simulink model "MPC_variants"  (R2026a)
settings: Solver=FixedStepAuto
settings Model: Creator=rayyu  LastModifiedBy=rayyu
settings RTWCC: SystemTargetFile=ert.tlc  Description=Embedded Coder
settings ERTTargetCC: GenerateSampleERTMain=on

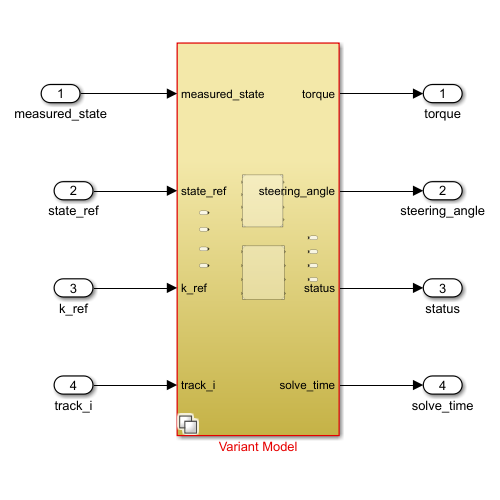
[thumbnail: Simulink's stored preview of the top-level diagram]
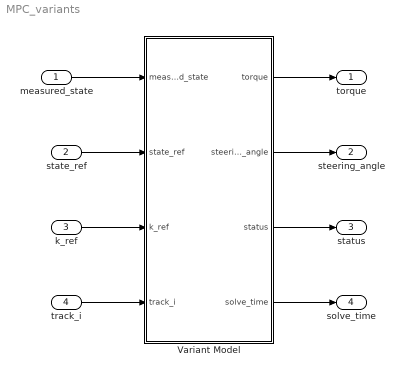
== system MPC_variants ==
  measured_state : Inport
  state_ref : Inport  Port=2
  k_ref : Inport  Port=3
  track_i : Inport  Port=4
  Variant Model : Subsystem  Variant=on
  torque : Outport
  steering_angle : Outport  Port=2
  status : Outport  Port=3
  solve_time : Outport  Port=4
  wires:
  measured_state/1 -> Variant Model/1(measured_state)
  state_ref/1 -> Variant Model/2(state_ref)
  k_ref/1 -> Variant Model/3(k_ref)
  track_i/1 -> Variant Model/4(track_i)
  Variant Model/1(torque) -> torque/1
  Variant Model/2(steering_angle) -> steering_angle/1
  Variant Model/3(status) -> status/1
  Variant Model/4(solve_time) -> solve_time/1

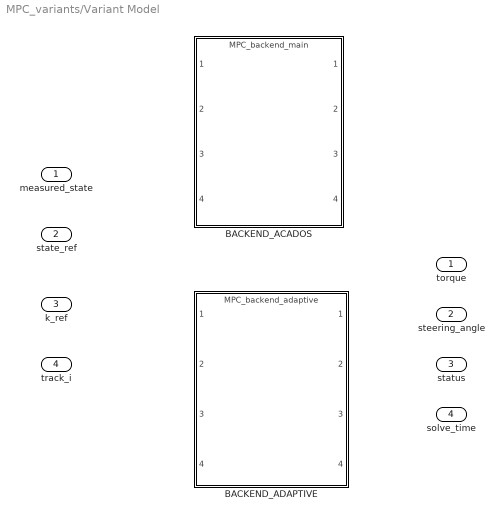
== system MPC_variants/Variant Model ==
  measured_state : Inport
  state_ref : Inport  Port=2
  k_ref : Inport  Port=3
  track_i : Inport  Port=4
  BACKEND_ACADOS : ModelReference  ModelNameDialog=MPC_backend_main.slx  SimulationMode=Normal  VariantControl=controllerParams.controller_backend == 1  ModelReferenceVersion=1.97
  BACKEND_ADAPTIVE : ModelReference  ModelNameDialog=MPC_backend_adaptive.slx  SimulationMode=Normal  VariantControl=controllerParams.controller_backend == 2  ModelReferenceVersion=1.48
  torque : Outport
  steering_angle : Outport  Port=2
  status : Outport  Port=3
  solve_time : Outport  Port=4
